simulink model "FractionalVoltage"  (R2015a)
settings: Solver=ode45  StartTime=0.0  StopTime=10  RelTol=1e-3
libraries: powerlib x12, simulink x2, powerlib_extras x1, re_lib x1
settings Model: Creator=user  LastModifiedBy=user

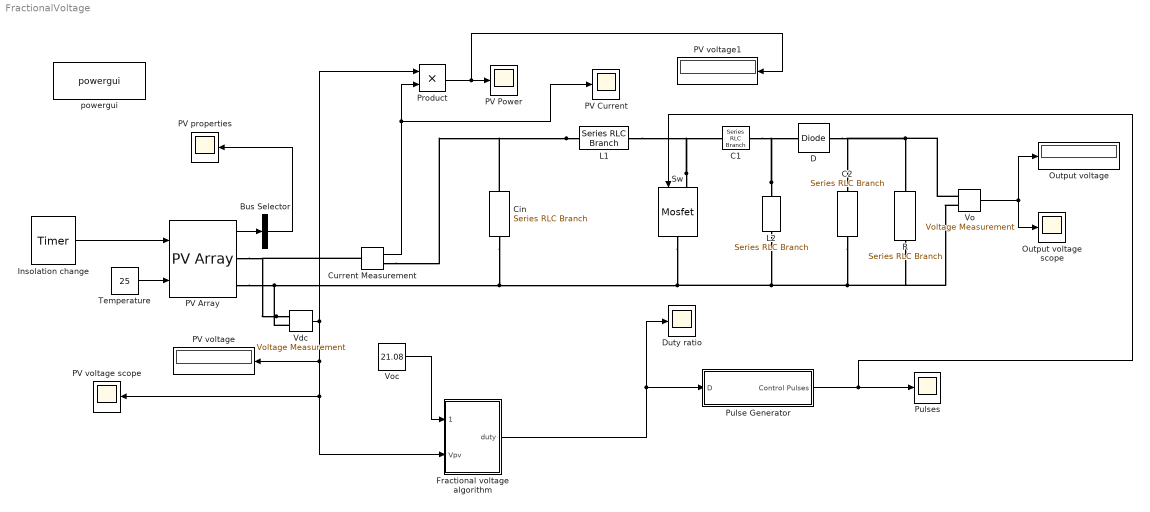
== system FractionalVoltage ==
  Bus Selector : BusSelector  OutputSignals=V_PV,I_PV  OutputAsBus=on
  C1 : powerlib/Elements/Series RLC Branch  LConnTagsString=__new0  RConnTagsString=__new0  BranchType=C  Resistance=100  Inductance=1e-3  SetiL0=off  InitialCurrent=0  Capacitance=20e-6  Setx0=off  InitialVoltage=0  Measurements=None
  C2 : powerlib/Elements/Series RLC Branch  LConnTagsString=__new0  RConnTagsString=__new0  BranchType=C  Resistance=1  Inductance=1e-3  SetiL0=off  InitialCurrent=0  Capacitance=150e-6  Setx0=off  InitialVoltage=0  Measurements=None
  Cin : powerlib/Elements/Series RLC Branch  LConnTagsString=__new0  RConnTagsString=__new0  BranchType=C  Resistance=1  Inductance=1e-3  SetiL0=off  InitialCurrent=0  Capacitance=440e-6  Setx0=off  InitialVoltage=0  Measurements=None
  Current Measurement : powerlib/Measurements/Current Measurement  PhasorSimulation=off  OutputType=Complex  PSBequivalent=0
  D : powerlib/Power Electronics/Diode  Ron=0.001  Lon=0  Vf=.05  IC=0  UseSnubber=off  Rs=500  Cs=250e-9  Measurements=off
  Duty ratio : Scope
      settings: ShowLegends=on  TimeRange=1  YMin=-138000  YMax=-117000
  Fractional voltage algorithm : Subsystem
  Insolation change : powerlib_extras/Control  Blocks/Timer  t="[0  5]"  e="[270   480]"
  L1 : powerlib/Elements/Series RLC Branch  LConnTagsString=__new0  RConnTagsString=__new0  BranchType=L  Resistance=1  Inductance=90e-6  SetiL0=off  InitialCurrent=0  Capacitance=1e-6  Setx0=off  InitialVoltage=0  Measurements=None
  L2 : powerlib/Elements/Series RLC Branch  LConnTagsString=__new0  RConnTagsString=__new0  BranchType=L  Resistance=1  Inductance=90e-6  SetiL0=off  InitialCurrent=0  Capacitance=1e-6  Setx0=off  InitialVoltage=0  Measurements=None
  Output voltage : Display
  Output voltage scope : Scope
      settings: ShowLegends=on  TimeRange=1  YMin=-1  YMax=2  SaveName=ScopeData3
  PV Array : re_lib/Solar/PV Array  Npar=9  Nser=4  PlotType=one module @ 25 deg.C & specified irradiances  S_vec=[270 480]  Temp_C_vec="[ 45 25  ]"  ModuleName=User-defined  PlotWhenSelected=on  Pm=20.1544  Ncell=36  Voc=21.17  Isc=1.26  Vm=17.08  Im=1.18  beta_Voc_pc=-0.2941  alpha_Isc_pc=0.0681  beta_Voc=-0.062261  alpha_Isc=0.00085806  IL=1.2621  I0=3.4157e-12  nI=0.85997  Rsh=849.2491  Rs=1.4265  BAL=on  Tc=1e-6  Tfilter=2e-5
  PV Current : Scope
      settings: ShowLegends=on  TimeRange=0.02  YMin=5.4263  YMax=5.4284  SaveName=ScopeData7  ScrollMode=on
  PV Power : Scope
      settings: ShowLegends=on  TimeRange=0.02  YMin=82  YMax=93  SaveName=ScopeData6  ScrollMode=on
  PV properties : Scope
      settings: ShowLegends=on  TimeRange=0.02  YMin=77.45762711864404  YMax=317.457627118644  ScrollMode=on
  PV voltage : Display
  PV voltage scope : Scope
      settings: TimeRange=1  YMin=0  YMax=500  SaveName=ScopeData5
  PV voltage1 : Display
  Product : Product
  Pulse Generator : Subsystem  mask{F=50e3}
      mask prompts: F "Carrier Frequency"
  Pulses : Scope
      settings: TimeRange=1  YMin=-1  YMax=2  SaveName=ScopeData4
  R : powerlib/Elements/Series RLC Branch  LConnTagsString=__new0  RConnTagsString=__new0  BranchType=R  Resistance=10  Inductance=1e-3  SetiL0=off  InitialCurrent=0  Capacitance=1e-6  Setx0=off  InitialVoltage=0  Measurements=None
  Sw : powerlib/Power Electronics/Mosfet  Ron=0.1  Lon=0  Rd=0.01  Vfd=0  IC=0  Rs=1e5  Cs=inf  Measurements=off
  Temperature : Constant  Value=25  VectorParams1D=off  SampleTime=2e-5
  "Vdc " : powerlib/Measurements/Voltage Measurement  Tag=PoWeRsYsTeMmEaSuReMeNt  PhasorSimulation=off  OutputType=Magnitude  PSBequivalent=0
  Vo : powerlib/Measurements/Voltage Measurement  PhasorSimulation=off  OutputType=Complex  PSBequivalent=0
  Voc : Constant  Value=21.08  VectorParams1D=off  SampleTime=2e-5
  powergui : powerlib/powergui  Priority=1  SimulationMode=Discrete  SolverType=Tustin/Backward Euler (TBE)  SampleTime=50e-6  frequency=50  SPID=on  DisableSnubberDevices=off  DisableRonSwitches=off  DisableVfSwitches=on  SwTol=0  DisplayEquations=off  Interpol=off  methode=off  Ts=0  FunctionMessages=off  echomessages=off  HookPort=off  EnableUseOfTLC=off  x0status=blocks  frequencyindice=0  Pbase=100e6  ErrMax=1e-4  Iterations=50  UnitsV=kV  UnitsW=MW  buscounter=0  RestoreLinks=warning  ResistiveCurrentMeasurement=off  Frange=[0:2:500]  Ylog=off  Xlog=on  ShowGrid=off  save=off  variable=ZData  structure=0  ZoomFFT=on  StartTime=0.0  cycles=1  DisplayStyle=1  fundamental=60  FreqAxis=off  MaxFrequency=1000  frequencyindicesteady=1  RmsSteady=1  display=off
  wires:
  PV Array/1 -> Bus Selector/1
  Vo/1 -> Output voltage scope/1, Output voltage/1
  Fractional voltage algorithm/1(duty) -> Duty ratio/1, Pulse Generator/1(D)
  Pulse Generator/1(Control Pulses) -> Sw/1, Pulses/1
  Bus Selector/1 -> PV properties/1
  Temperature/1 -> PV Array/2
  "Vdc "/1 -> PV voltage/1, Fractional voltage algorithm/2(Vpv), PV voltage scope/1, Product/1
  Product/1 -> PV voltage1/1, PV Power/1
  Current Measurement/1 -> PV Current/1, Product/2
  Insolation change/1 -> PV Array/1
  Voc/1 -> Fractional voltage algorithm/1(VocREF)
  connections:
  "Vdc "/LConn2 -- PV Array/RConn2 -- Cin/RConn1 -- Sw/RConn1 -- L2/RConn1 -- C2/RConn1 -- Vo/LConn2 -- R/RConn1
  Sw/LConn1 -- L1/RConn1 -- C1/LConn1
  Vo/LConn1 -- R/LConn1 -- C2/LConn1 -- D/RConn1
  L2/LConn1 -- C1/RConn1 -- D/LConn1
  L1/LConn1 -- Current Measurement/RConn1 -- Cin/LConn1
  "Vdc "/LConn1 -- Current Measurement/LConn1 -- PV Array/RConn1

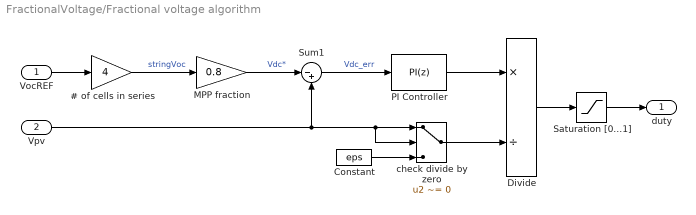
== system FractionalVoltage/Fractional voltage algorithm ==
  VocREF : Inport  OutDataTypeStr=double  PortDimensions=1  SampleTime=[0.0001,0]
  Vpv : Inport  Port=2  OutDataTypeStr=double  PortDimensions=1  SampleTime=[0.0001,0]
  # of cells in series : Gain  Gain=4
  Constant : Constant  Value=eps
  Divide : Product  Inputs=*/
  MPP fraction : Gain  Gain=0.8
  PI Controller : simulink/Continuous/PID Controller  Controller=PI  TimeDomain=Discrete-time  SampleTime=1e-4  IntegratorMethod=Forward Euler  FilterMethod=Forward Euler  Form=Parallel  UseFilter=on  ControllerParametersSource=internal  P=1  I=250  D=0  N=100  InitialConditionSource=internal  InitialConditionForIntegrator=186.4  InitialConditionForFilter=0  ExternalReset=none  ZeroCross=off  LimitOutput=off  UpperSaturationLimit=1  LowerSaturationLimit=0  LinearizeAsGain=off  AntiWindupMode=none  Kb=1  TrackingMode=off  Kt=1  PParamMin=[]  PParamMax=[]  IParamMin=[]  IParamMax=[]  DParamMin=[]  DParamMax=[]  NParamMin=[]  NParamMax=[]  KbParamMin=[]  KbParamMax=[]  KtParamMin=[]  KtParamMax=[]  POutMin=[]  POutMax=[]  IOutMin=[]  IOutMax=[]  DOutMin=[]  DOutMax=[]  NOutMin=[]  NOutMax=[]  KbOutMin=[]  KbOutMax=[]  KtOutMin=[]  KtOutMax=[]  IntegratorOutMin=[]  IntegratorOutMax=[]  FilterOutMin=[]  FilterOutMax=[]  SumOutMin=[]  SumOutMax=[]  SumI1OutMin=[]  SumI1OutMax=[]  SumI2OutMin=[]  SumI2OutMax=[]  SumI3OutMin=[]  SumI3OutMax=[]  SumDOutMin=[]  SumDOutMax=[]  SaturationOutMin=[]  SaturationOutMax=[]  IntegratorContinuousStateAttributes=''  IntegratorStateMustResolveToSignalObject=off  IntegratorRTWStateStorageClass=Auto  FilterContinuousStateAttributes=''  FilterStateMustResolveToSignalObject=off  FilterRTWStateStorageClass=Auto  DifferentiatorICPrevScaledInput=0  DifferentiatorOutMin=[]  DifferentiatorOutMax=[]
  Saturation [0...1] : Saturate  UpperLimit=1  LowerLimit=0
  Sum1 : Sum  Inputs=|-+
  check divide by zero : Switch  Criteria=u2 ~= 0
  duty : Outport  OutDataTypeStr=double  PortDimensions=1  SampleTime=[0.0001,0]
  wires:
  Saturation [0...1]/1 -> duty/1
  VocREF/1 -> # of cells in series/1
  Divide/1 -> Saturation [0...1]/1
  PI Controller/1 -> Divide/1
  # of cells in series/1 -> MPP fraction/1  "stringVoc"
  MPP fraction/1 -> Sum1/1  "Vdc*"
  Sum1/1 -> PI Controller/1  "Vdc_err"
  Vpv/1 -> check divide by zero/2, check divide by zero/1, Sum1/2
  check divide by zero/1 -> Divide/2
  Constant/1 -> check divide by zero/3

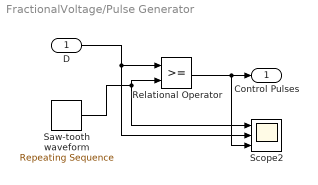
== system FractionalVoltage/Pulse Generator ==
  D : Inport
  Relational Operator : RelationalOperator  OutDataTypeStr=boolean
  Saw-tooth waveform : simulink/Sources/Repeating Sequence  rep_seq_t=[0 0.5 1]/F  rep_seq_y=[0 1 0]
  Scope2 : Scope  NumInputPorts=3
      settings: TimeRange=0.004  YMin=5.55112e-017~0.7~0  YMax=1~0.7~1  SaveName=ScopeData2
  Control Pulses : Outport
  wires:
  Saw-tooth waveform/1 -> Relational Operator/2, Scope2/1
  Relational Operator/1 -> Scope2/3, Control Pulses/1
  D/1 -> Relational Operator/1, Scope2/2
